simulink model "gain_calculation"  (R2020b)
settings: Solver=FixedStepAuto  StartTime=0.0  StopTime=stop_time  RelTol=1e-3
settings Model: Creator=conno  LastModifiedBy=tyler
settings DataIOCC: ReturnWorkspaceOutputs=off
settings OptimizationCC: DefaultParameterBehavior=Inlined
settings ModelReferenceCC: ModelReferenceNumInstancesAllowed=Single

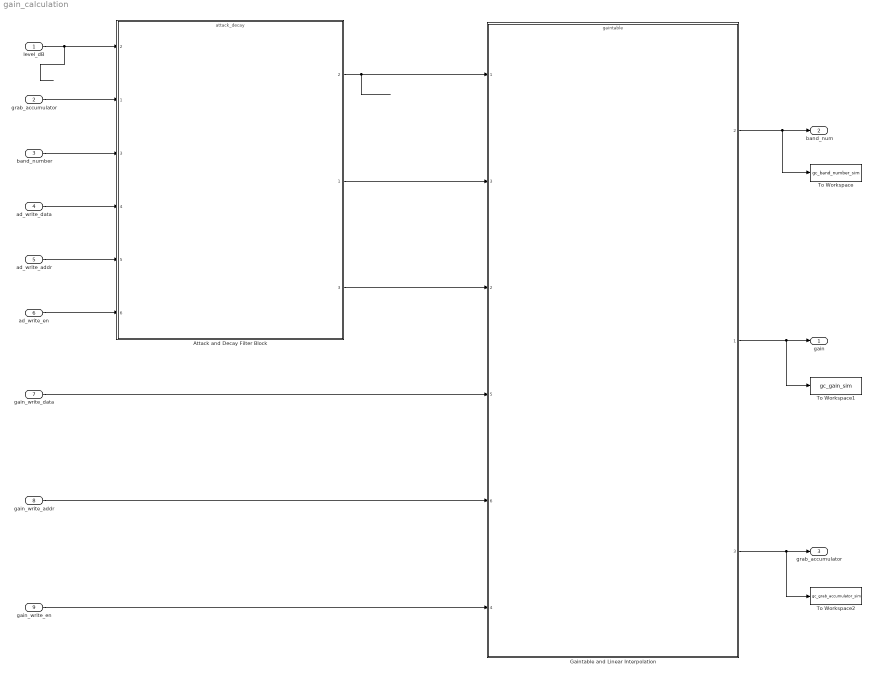
== system gain_calculation ==
  level_dB : Inport
  grab_accumulator : Inport  Port=2
  band_number : Inport  Port=3
  ad_write_data : Inport  Port=4  OutDataTypeStr=ad_coeff_type
  ad_write_addr : Inport  Port=5  OutDataTypeStr=uint8
  ad_write_en : Inport  Port=6  OutDataTypeStr=boolean
  gain_write_data : Inport  Port=7  OutDataTypeStr=gain_coeff_type
  gain_write_addr : Inport  Port=8  OutDataTypeStr=uint8
  gain_write_en : Inport  Port=9  OutDataTypeStr=boolean
  Attack and Decay Filter Block : ModelReference  ModelNameDialog=attack_decay.slx  SimulationMode=Normal  ModelReferenceVersion=2.93
      settings: PortSchema="{\"entries\":[{\"content\":{\"sides\":[{\"content\":{\"connectorIds\":[\"In2\",\"In1\",\"In3\",\"In4\",\"In5\",\"In6\"]},\"type\":\"ConnectorPlacement.EquallySpacedRectSide\",\"uuid\":\"fcf0b3b6-5812-4ef4-90f3-cd4a0efc9468\"},{\"content\":{\"connectorIds\":[\"Out2\",\"Out1\",\"Out3\"],\"side\":\"RIGHT\"},\"type\":\"ConnectorPlacement.EquallySpacedRectSide\",\"uuid\":\"ac266780-5249-46a9-8938-d8ecb069819a\"},{\"content\":{\"connectorIds\":[],\"side\":\"TOP\"},\"type\":\"ConnectorPlacement.EquallySpacedRectSide\",\"uuid\":\"cfc157a2-de57-4f22-8943-db0b5873c905\"},{\"content\":{\"connectorIds\":[],\"side\":\"HIDDEN\"},\"type\":\"ConnectorPlacement.EquallySpacedRectSide\",\"uuid\":\"ad99eb54-0bd3-4d9e-8c95-caad9c131696\"}]},\"type\":\"ConnectorPlacement.EquallySpacedConnector\",\"uuid\":\"9e8a55f5-cdb7-43a1-a9e8-10d3297cead2\"}],\"packageUris\":[\"http://schema.mathworks.com/mf0/Connector/R2020b\"],\"version\":\"1.0\"}"
  Gaintable and Linear Interpolation : ModelReference  ModelNameDialog=gaintable.slx  SimulationMode=Normal  ModelReferenceVersion=2.76
      settings: PortSchema="{\"entries\":[{\"content\":{\"sides\":[{\"content\":{\"connectorIds\":[\"In1\",\"In3\",\"In2\",\"In5\",\"In6\",\"In4\"]},\"type\":\"ConnectorPlacement.EquallySpacedRectSide\",\"uuid\":\"fcf0b3b6-5812-4ef4-90f3-cd4a0efc9468\"},{\"content\":{\"connectorIds\":[\"Out2\",\"Out1\",\"Out3\"],\"side\":\"RIGHT\"},\"type\":\"ConnectorPlacement.EquallySpacedRectSide\",\"uuid\":\"ac266780-5249-46a9-8938-d8ecb069819a\"},{\"content\":{\"connectorIds\":[],\"side\":\"TOP\"},\"type\":\"ConnectorPlacement.EquallySpacedRectSide\",\"uuid\":\"cfc157a2-de57-4f22-8943-db0b5873c905\"},{\"content\":{\"connectorIds\":[],\"side\":\"HIDDEN\"},\"type\":\"ConnectorPlacement.EquallySpacedRectSide\",\"uuid\":\"ad99eb54-0bd3-4d9e-8c95-caad9c131696\"}]},\"type\":\"ConnectorPlacement.EquallySpacedConnector\",\"uuid\":\"9e8a55f5-cdb7-43a1-a9e8-10d3297cead2\"}],\"packageUris\":[\"http://schema.mathworks.com/mf0/Connector/R2020b\"],\"version\":\"1.0\"}"
  To Workspace : ToWorkspace  VariableName=gc_band_number_sim  SaveFormat=Timeseries  SampleTime=-1
  To Workspace1 : ToWorkspace  VariableName=gc_gain_sim  SaveFormat=Timeseries  SampleTime=-1
  To Workspace2 : ToWorkspace  VariableName=gc_grab_accumulator_sim  SaveFormat=Timeseries  SampleTime=-1
  gain : Outport
  band_num : Outport  Port=2
  "grab_accumulator " : Outport  Port=3  PortDimensions=1
  wires:
  ad_write_data/1 -> Attack and Decay Filter Block/4
  ad_write_addr/1 -> Attack and Decay Filter Block/5
  ad_write_en/1 -> Attack and Decay Filter Block/6
  Gaintable and Linear Interpolation/2 -> To Workspace/1, band_num/1
  Gaintable and Linear Interpolation/1 -> To Workspace1/1, gain/1
  gain_write_en/1 -> Gaintable and Linear Interpolation/4
  gain_write_addr/1 -> Gaintable and Linear Interpolation/6
  gain_write_data/1 -> Gaintable and Linear Interpolation/5
  Gaintable and Linear Interpolation/3 -> To Workspace2/1, "grab_accumulator "/1
  Attack and Decay Filter Block/3 -> Gaintable and Linear Interpolation/2
  Attack and Decay Filter Block/1 -> Gaintable and Linear Interpolation/3
  Attack and Decay Filter Block/2 -> Gaintable and Linear Interpolation/1
  level_dB/1 -> Attack and Decay Filter Block/2
  grab_accumulator/1 -> Attack and Decay Filter Block/1
  band_number/1 -> Attack and Decay Filter Block/3
